simulink model "PlantStateEquations_abc"  (R2018a)
settings: Solver=VariableStepAuto  StartTime=0.0  StopTime=2  FixedStep=Ts_sim  RelTol=1e-3
values from neighbouring files (symbols this model uses):
  ess = {}    [PlantStateEquations_abc_Script.m]
  ibini = 0    [PlantStateEquations_abc_Script.m]
  igaaini = 0    [PlantStateEquations_abc_Script.m]
  igabini = 0    [PlantStateEquations_abc_Script.m]
  igacini = 0    [PlantStateEquations_abc_Script.m]
  mb = 1    [PlantStateEquations_abc_Script.m]
  systemBase = {}    [PlantStateEquations_abc_Script.m]
  vb = ess.Udc    [PlantStateEquations_abc_Script.m]
  vdcini = ess.Udc    [PlantStateEquations_abc_Script.m]
libraries: powerlib x3, pwrsysVSrc x2, pwrsysBasic x1
settings Model: Creator=daniemot  LastModifiedBy=daniemot

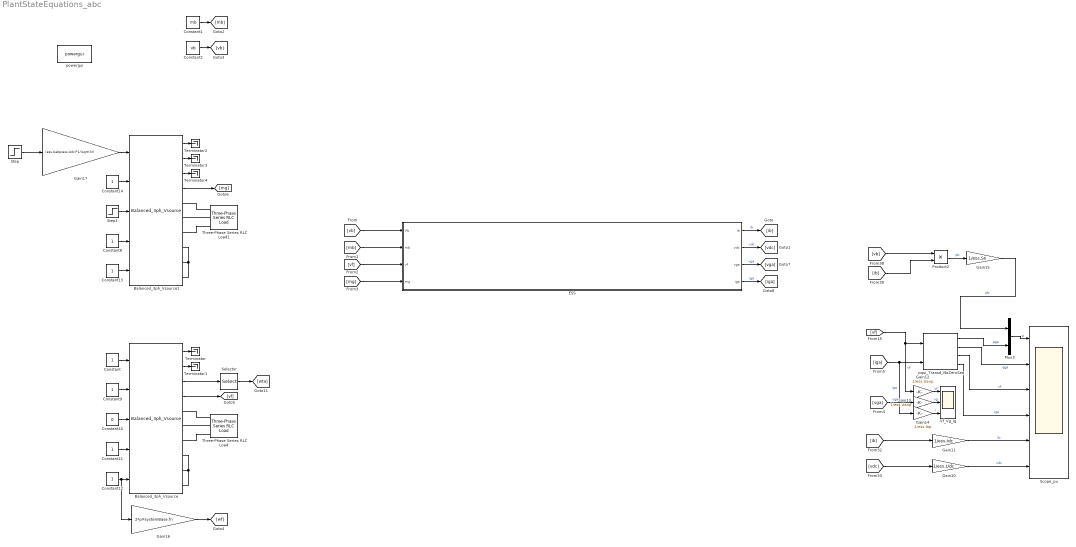
== system PlantStateEquations_abc ==
  Balanced_3ph_Vsource : pwrsysVSrc/Balanced_3ph_Vsource  BaseAmp=ess.Uanp  fn=systemBase.fn  AmpIni=ess.Uanp  SeqIni=1  AngIni=0  FIni=systemBase.fn  HarmIni=1
      settings: SourceProductName=NTNU Power Systems
  Balanced_3ph_Vsource1 : pwrsysVSrc/Balanced_3ph_Vsource  BaseAmp=1  fn=systemBase.fn  AmpIni=1  SeqIni=1  AngIni=0  FIni=systemBase.fn  HarmIni=1
      settings: SourceProductName=NTNU Power Systems
  Constant{,8..9,11..14} (7 alike) : Constant
  Constant1 : Constant  Value=mb
  Constant10 : Constant  Value=0
  Constant2 : Constant  Value=vb
  ESS : Subsystem  mask{Rb=ess.LCL.R1, Lb=ess.LCL.L1, R1=ess.LCL.R1, L1=ess.LCL.L1, Cdc=ess.Cdc, Rdc=100e3}
      mask prompts: Rb "Resistance, Rb [Ohm]"; Lb "Inductance, Lb [H]"; R1 "Main reactor resistance, R1 [Ohm]"; L1 "Main Reactor inductance, L1 [H]"; Cdc "DC-link capacitance, Cdc [F]"; Rdc "DC-link shunt resistance, Rdc [Ohm]"
      mask DialogControl Container4 Prompt: DC-DC Converter
      mask DialogControl Container3 Prompt: AC-DC Converter
      mask Display: image('L_BC_C_GC_L.png');
  Gain10 : Gain  Gain=1/ess.Udc
  Gain11 : Gain  Gain=1/ess.Idc
  Gain12 : Gain  Gain=1/ess.Uanp
  Gain13 : Gain  Gain=1/ess.Uanp
  Gain14 : Gain  Gain=1/ess.Iap
  Gain15 : Gain  Gain=1/ess.Sn
  Gain16 : Gain  Gain=2*pi*systemBase.fn
  Gain17 : Gain  Gain=(ess.Uabp/ess.Udc)*1/(sqrt(3))
  Mux3 : Mux  Inputs=2
  Product2 : Product
  Scope_pu : Scope  NumInputPorts=6
  Selector : Selector  InputPortWidth=3  IndexOptions=Index vector (dialog)  Indices=[1]  OutputSizes=1
  Step : Step  Time=0.5  Before=1  After=1.1  SampleTime=0
  Step1 : Step  After=10  SampleTime=0
  Terminator{,1..4} (5 alike) : Terminator
  Three-Phase Series RLC Load : powerlib/Elements/Three-Phase Series RLC Load  LConnTagsString=A|B|C  Configuration=Y (grounded)  NominalVoltage=ess.Un  Vabc=[1e3 1e3 1e3]  Vabcp=[1e3 1e3 1e3]  NominalFrequency=systemBase.fn  UnbalancedPower=off  ActivePower=1000  InductivePower=0  CapacitivePower=0  Pabc=[10e3 9e3 11e3]  QLabc=[100 90 110]  QCabc=[100 90 110]  Pabcp=[10e3 9e3 11e3]  QLabcp=[100 90 110]  QCabcp=[100 90 110]  Measurements=None  LoadType=constant Z
  Three-Phase Series RLC Load1 : powerlib/Elements/Three-Phase Series RLC Load  LConnTagsString=A|B|C  Configuration=Y (grounded)  NominalVoltage=ess.Un  Vabc=[1e3 1e3 1e3]  Vabcp=[1e3 1e3 1e3]  NominalFrequency=systemBase.fn  UnbalancedPower=off  ActivePower=1000  InductivePower=0  CapacitivePower=0  Pabc=[10e3 9e3 11e3]  QLabc=[100 90 110]  QCabc=[100 90 110]  Pabcp=[10e3 9e3 11e3]  QLabcp=[100 90 110]  QCabcp=[100 90 110]  Measurements=None  LoadType=constant Z
  Vf_Vg_Ig : Scope  NumInputPorts=3
  powergui : powerlib/powergui  Priority=1  SimulationMode=Discrete  SampleTime=50e-6  frequency=60  Iterations=50  frequencyindice=60  Pbase=100e6  ErrMax=1e-4  UnitsV=kV  UnitsW=MW  buscounter=0  FunctionMessages=off  echomessages=off  EnableUseOfTLC=off  CurrentSourceSwitches=off  DisableSnubberDevices=off  DisableRonSwitches=off  DisableVfSwitches=off  DisplayEquations=off  SolverType=Tustin/Backward Euler (TBE)  Interpol=off  ExternalGateDelay=off  methode=off  Ts=100  x0status=blocks  SPID=off  SwTol=0  HookPort=off  RestoreLinks=warning  ResistiveCurrentMeasurement=off  Frange=[0:2:500]  Ylog=off  Xlog=on  ShowGrid=off  save=off  variable=ZData  structure=0  ZoomFFT=off  StartTime=0.0  cycles=1  DisplayStyle=1  fundamental=60  FreqAxis=off  MaxFrequency=1000  frequencyindicesteady=1  RmsSteady=1  display=off
  pqui_Transd_NoZeroSeq : pwrsysBasic/pqui_Transd_NoZeroSeq  Sn=ess.Sn  Uanp=ess.Uanp  Iap=ess.Iap
      settings: SourceProductName=NTNU Power Systems
  wires:
  Constant1/1 -> [mb]
  Constant2/1 -> [vb]
  Product2/1 -> Gain15/1  "pb"
  [vb] -> Product2/1
  [ib] -> Product2/2
  Gain15/1 -> Mux3/1  "pb"
  Constant/1 -> Balanced_3ph_Vsource/1
  Constant9/1 -> Balanced_3ph_Vsource/2
  Constant10/1 -> Balanced_3ph_Vsource/3
  Constant11/1 -> Balanced_3ph_Vsource/4
  Constant12/1 -> Gain16/1, Balanced_3ph_Vsource/5
  Balanced_3ph_Vsource/4 -> [vf]
  Balanced_3ph_Vsource/1 -> Terminator/1
  Balanced_3ph_Vsource/2 -> Terminator1/1
  Balanced_3ph_Vsource/3 -> Selector/1
  Gain16/1 -> [wf]
  Selector/1 -> [wta]
  Constant8/1 -> Balanced_3ph_Vsource1/4
  Constant13/1 -> Balanced_3ph_Vsource1/5
  Step1/1 -> Balanced_3ph_Vsource1/3
  Constant14/1 -> Balanced_3ph_Vsource1/2
  Balanced_3ph_Vsource1/2 -> Terminator3/1
  Gain17/1 -> Balanced_3ph_Vsource1/1
  Balanced_3ph_Vsource1/1 -> Terminator2/1
  Balanced_3ph_Vsource1/3 -> Terminator4/1
  [vf] -> Gain12/1, pqui_Transd_NoZeroSeq/1  "vf"
  [iga] -> Gain14/1, pqui_Transd_NoZeroSeq/2  "iga"
  Step/1 -> Gain17/1
  pqui_Transd_NoZeroSeq/1 -> Mux3/2  "pga"
  pqui_Transd_NoZeroSeq/2 -> Scope_pu/2  "qga"
  pqui_Transd_NoZeroSeq/3 -> Scope_pu/3  "vf"
  pqui_Transd_NoZeroSeq/4 -> Scope_pu/4  "iga"
  [vdc] -> Gain10/1
  Gain10/1 -> Scope_pu/6  "vdc"
  Gain11/1 -> Scope_pu/5  "ib"
  [ib] -> Gain11/1
  Mux3/1 -> Scope_pu/1  "p"
  [vga] -> Gain13/1  "vga"
  Gain12/1 -> Vf_Vg_Ig/1  "vf"
  Gain13/1 -> Vf_Vg_Ig/2  "vg"
  Gain14/1 -> Vf_Vg_Ig/3  "i"
  [mb] -> ESS/2(mb)
  ESS/1(ib) -> [ib]  "ib"
  ESS/2(vdc) -> [vdc]  "vdc"
  [vb] -> ESS/1(Vb)
  [vf] -> ESS/3(vf)
  Balanced_3ph_Vsource1/4 -> [mg]
  [mg] -> ESS/4(mg)
  ESS/3(vga) -> [vga]  "vga"
  ESS/4(iga) -> [iga]  "iga"
  connections:
  Balanced_3ph_Vsource/RConn6 -- Balanced_3ph_Vsource/RConn4 -- Balanced_3ph_Vsource/RConn5
  Three-Phase Series RLC Load/LConn1 -- Balanced_3ph_Vsource/RConn1
  Three-Phase Series RLC Load/LConn2 -- Balanced_3ph_Vsource/RConn2
  Three-Phase Series RLC Load/LConn3 -- Balanced_3ph_Vsource/RConn3
  Balanced_3ph_Vsource1/RConn5 -- Balanced_3ph_Vsource1/RConn6 -- Balanced_3ph_Vsource1/RConn4
  Three-Phase Series RLC Load1/LConn2 -- Balanced_3ph_Vsource1/RConn2
  Three-Phase Series RLC Load1/LConn1 -- Balanced_3ph_Vsource1/RConn1
  Three-Phase Series RLC Load1/LConn3 -- Balanced_3ph_Vsource1/RConn3

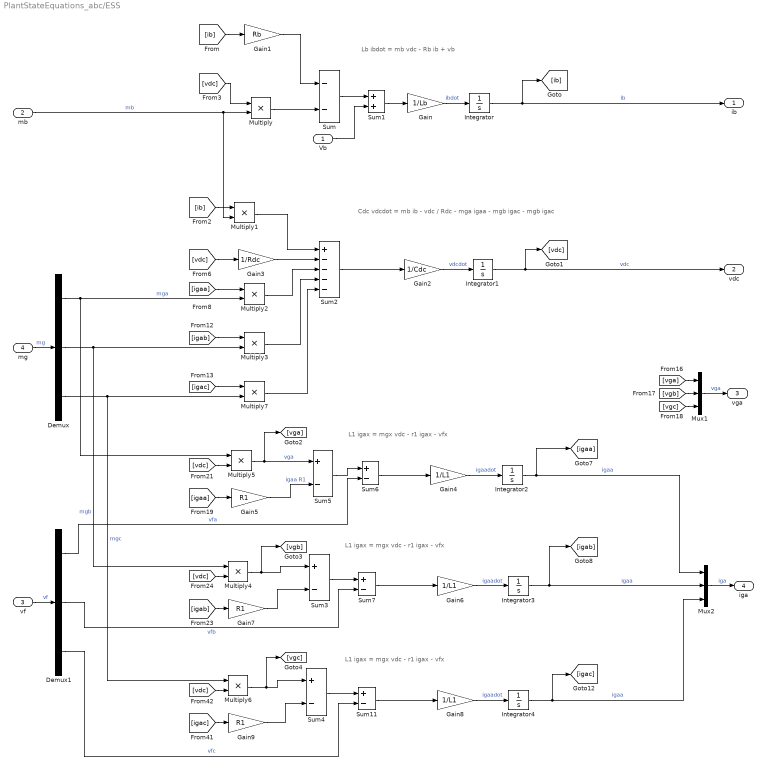
== system PlantStateEquations_abc/ESS ==
  note: Lb ibdot = mb vdc - Rb ib + vb
  note: Cdc vdcdot = mb ib - vdc / Rdc - mga igaa - mgb igac - mgb igac
  note: L1 igax = mgx vdc - r1 igax - vfx
  note: L1 igax = mgx vdc - r1 igax - vfx
  note: L1 igax = mgx vdc - r1 igax - vfx
  Vb : Inport
  mb : Inport  Port=2
  vf : Inport  Port=3
  mg : Inport  Port=4
  Demux : Demux  Outputs=3
  Demux1 : Demux  Outputs=3
  Gain : Gain  Gain=1/Lb
  Gain1 : Gain  Gain=Rb
  Gain2 : Gain  Gain=1/Cdc
  Gain3 : Gain  Gain=1/Rdc
  Gain4 : Gain  Gain=1/L1
  Gain5 : Gain  Gain=R1
  Gain6 : Gain  Gain=1/L1
  Gain7 : Gain  Gain=R1
  Gain8 : Gain  Gain=1/L1
  Gain9 : Gain  Gain=R1
  Integrator : Integrator  InitialCondition=ibini
  Integrator1 : Integrator  InitialCondition=vdcini
  Integrator2 : Integrator  InitialCondition=igaaini
  Integrator3 : Integrator  InitialCondition=igabini
  Integrator4 : Integrator  InitialCondition=igacini
  Multiply{,1..7} (8 alike) : Product
  Mux1 : Mux  Inputs=3
  Mux2 : Mux  Inputs=3
  Sum : Sum  Inputs=--
  Sum1 : Sum
  Sum{3..7,11} (6 alike) : Sum  Inputs=+-
  Sum2 : Sum  Inputs=+----
  ib : Outport
  vdc : Outport  Port=2
  vga : Outport  Port=3
  iga : Outport  Port=4
  wires:
  mb/1 -> Multiply1/2, Multiply/2  "mb"
  Gain1/1 -> Sum/1
  Integrator4/1 -> [igac], Mux2/3  "igaa"
  Multiply6/1 -> [vgc], Sum4/1
  Gain9/1 -> Sum4/2
  Gain2/1 -> Integrator1/1  "vdcdot"
  [vdc] -> Multiply/1
  Demux1/3 -> Sum11/2  "vfc"
  Multiply4/1 -> [vgb], Sum3/1
  Gain6/1 -> Integrator3/1  "igaadot"
  [igab] -> Gain7/1
  Sum5/1 -> Sum6/1
  Multiply7/1 -> Sum2/5
  Sum6/1 -> Gain4/1
  [igaa] -> Multiply2/1
  Multiply5/1 -> [vga], Sum5/1  "vga"
  Gain7/1 -> Sum3/2
  Sum4/1 -> Sum11/1
  Sum7/1 -> Gain6/1
  [ib] -> Gain1/1
  Gain3/1 -> Sum2/2
  [igaa] -> Gain5/1
  Gain/1 -> Integrator/1  "ibdot"
  Sum3/1 -> Sum7/1
  Demux1/1 -> Sum6/2  "vfa"
  Demux1/2 -> Sum7/2  "vfb"
  Multiply2/1 -> Sum2/3
  Integrator2/1 -> [igaa], Mux2/1  "igaa"
  Integrator/1 -> [ib], ib/1  "ib"
  [igab] -> Multiply3/1
  Multiply1/1 -> Sum2/1
  Demux/3 -> Multiply6/1, Multiply7/2  "mgc"
  Multiply3/1 -> Sum2/4
  [vdc] -> Gain3/1
  [vdc] -> Multiply4/2
  Sum/1 -> Sum1/1
  Multiply/1 -> Sum/2
  [vdc] -> Multiply5/2
  Gain4/1 -> Integrator2/1  "igaadot"
  Sum1/1 -> Gain/1
  Gain5/1 -> Sum5/2  "igaa R1"
  Vb/1 -> Sum1/2
  [igac] -> Multiply7/1
  Sum11/1 -> Gain8/1
  Integrator3/1 -> [igab], Mux2/2  "igaa"
  Gain8/1 -> Integrator4/1  "igaadot"
  Demux/2 -> Multiply4/1, Multiply3/2  "mgb"
  Demux/1 -> Multiply5/1, Multiply2/2  "mga"
  [ib] -> Multiply1/1
  [vdc] -> Multiply6/2
  [igac] -> Gain9/1
  Sum2/1 -> Gain2/1
  Integrator1/1 -> [vdc], vdc/1  "vdc"
  Mux1/1 -> vga/1  "vga"
  [vgc] -> Mux1/3
  [vga] -> Mux1/1
  [vgb] -> Mux1/2
  Mux2/1 -> iga/1  "iga"
  mg/1 -> Demux/1  "mg"
  vf/1 -> Demux1/1  "vf"
